simulink model "Proyecto"  (R2023b)
settings: Solver=FixedStepDiscrete  StartTime=0.0  StopTime=100  FixedStep=0.01  MaxStep=0.01  RelTol=1e-3  EnableMultiTasking=on
model workspace (MAT data in the model file):
  d = 0.223
libraries: robotalgslib x1
settings Model: ExtModeTrigDuration=2  Creator=Manuel  LastModifiedBy=Manuel
settings OptimizationCC: EnhancedBackFolding=on  PassReuseOutputArgsAs=Individual arguments  ZeroExternalMemoryAtStartup=off  ZeroInternalMemoryAtStartup=off  MaxStackSize=64  OptimizeBlockOrder=speed  DifferentSizesBufferReuse=on  EfficientTunableParamExpr=on
settings DebuggingCC: AlgebraicLoopMsg=none  ParameterTunabilityLossMsg=error
settings HardwareCC: ProdBitPerInt=16  ProdBitPerPointer=16  ProdBitPerSizeT=16  ProdBitPerPtrDiffT=16  ProdLargestAtomicFloat=None  ProdWordSize=8  ProdHWDeviceType=Atmel->AVR
settings SFSimCC: MATLABDynamicMemAlloc=off
settings RTWCC: Description=Embedded Coder  SystemTargetFile=ert.tlc  HardwareBoard=Arduino Mega 2560  TemplateMakefile=ert_default_tmf  Toolchain=Arduino AVR  BuildConfiguration=Faster Runs
settings CodeAppCC: ForceParamTrailComments=on  IgnoreCustomStorageClasses=off  OperatorAnnotations=on  SimulinkDataObjDesc=on  SFDataObjDesc=on  InsertBlockDesc=on
settings ERTTargetCC: SupportContinuousTime=on  SupportVariableSizeSignals=on  ExtModeTransport=3  ExtModeStaticAlloc=on  ExtModeAutomaticAllocSize=off  ExtModeStaticAllocSize=2048  ExtModeMexFile=ext_xcp  ExtModeIntrfLevel=Level2 - Open

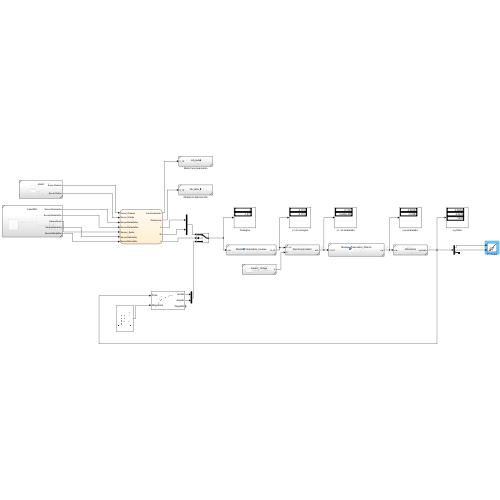
[thumbnail: Simulink's stored preview of the top-level diagram]
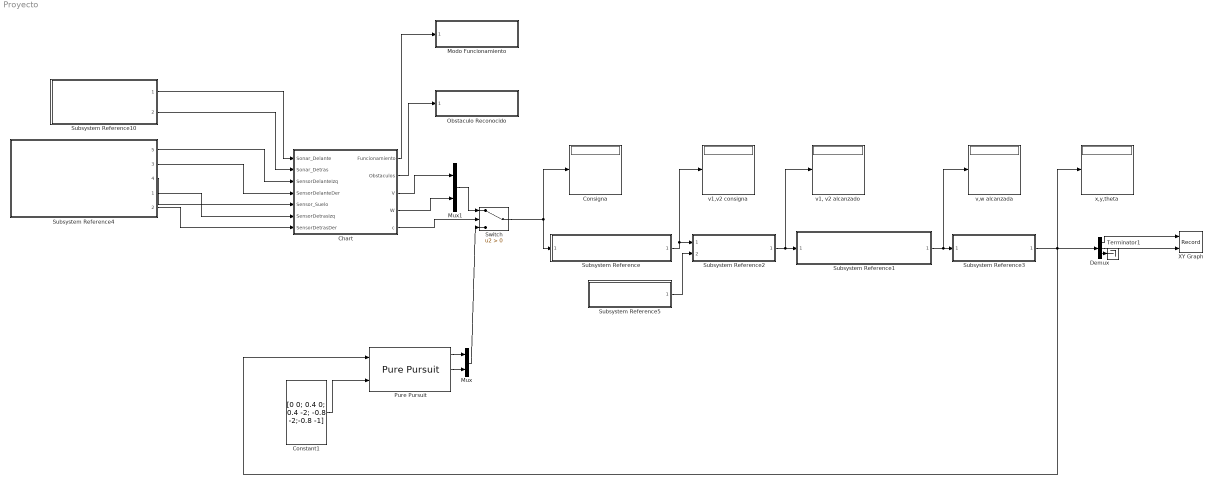
== system Proyecto ==
  Chart : Stateflow chart  TreatAsAtomicUnit=on
      settings: PortSchema="{\"entries\":[{\"content\":{\"sides\":[{\"content\":{\"connectorIds\":[\"In1\",\"In2\",\"In3\",\"In4\",\"In5\",\"In6\",\"In7\"]},\"type\":\"ConnectorPlacement.EquallySpacedRectSide\",\"uuid\":\"4f2d59c3-0ad9-459c-b559-bc93b323e865\"},{\"content\":{\"connectorIds\":[\"Out1\",\"Out2\",\"Out4\",\"Out5\",\"Out3\"],\"side\":\"RIGHT\"},\"type\":\"ConnectorPlacement.EquallySpacedRectSide\",\"uuid\":\"713f980b-cafd-4d08-9887-886c0fa4174d\"},{\"content\":{\"side\":\"TOP\"},\"type\":\"ConnectorPlacement.EquallySpacedRectSide\",\"uuid\":\"6d2f14ce-a548-4b18-94d2-b32a2277c49c\"},{\"content\":{\"side\":\"BOTTOM\"},\"type\":\"ConnectorPlacement.EquallySpacedRectSide\",\"uuid\":\"144d8ec0-92fa-4068-8952-ba018721fcc9\"}]},\"type\":\"ConnectorPlacement.EquallySpacedConnector\",\"uuid\":\"e616e035-6f8b-4bd0-b456-c7d21c102a60\"}],\"packageUris\":[\"http://schema.mathworks.com/mf0/Connector/R2020b\"],\"version\":\"1.0\"}"
  Consigna : Display
  Constant1 : Constant  Value=[0 0; 0.4 0; 0.4 -2; -0.8 -2;-0.8 -1]
  Demux : Demux  Outputs=3
  Modo Funcionamiento : Subsystem  ReferencedSubsystem=Lib_leds
  Mux : Mux  Inputs=2
  Mux1 : Mux  Inputs=2
  Obstaculo Reconocido : Subsystem  ReferencedSubsystem=Lib_leds_2
  Pure Pursuit : robotalgslib/Pure Pursuit  DesiredLinearVelocity=0.3  MaxAngularVelocity=pi/2  LookaheadDistance=0.22  TargetDirPort=on  SimulateUsing=Code generation
      settings: LibrarySourceBlock=navlib/Control Algorithms/Pure Pursuit
  Subsystem Reference : Subsystem  ReferencedSubsystem=Modelo_Cinematico_Inverso
  Subsystem Reference1 : Subsystem  ReferencedSubsystem=Modelo_Cinematico_Directo
  Subsystem Reference10 : Subsystem  ReferencedSubsystem=sonar
  Subsystem Reference2 : Subsystem  ReferencedSubsystem=PieroControladoV
  Subsystem Reference3 : Subsystem  ReferencedSubsystem=Odometria
  Subsystem Reference4 : Subsystem  ReferencedSubsystem=LaserMm
      settings: PortSchema="{\"entries\":[{\"content\":{\"sides\":[{\"content\":{},\"type\":\"ConnectorPlacement.EquallySpacedRectSide\",\"uuid\":\"00a5621a-91c8-4fa0-83fa-79bbc13aa011\"},{\"content\":{\"connectorIds\":[\"Out5\",\"Out3\",\"Out4\",\"Out1\",\"Out2\"],\"side\":\"RIGHT\"},\"type\":\"ConnectorPlacement.EquallySpacedRectSide\",\"uuid\":\"6fca1f99-4dc9-459c-b010-38f5feebdec4\"},{\"content\":{\"side\":\"TOP\"},\"type\":\"ConnectorPlacement.EquallySpacedRectSide\",\"uuid\":\"4ca4df48-19f6-46c7-814a-4f1771035d4e\"}]},\"type\":\"ConnectorPlacement.EquallySpacedConnector\",\"uuid\":\"c2dd7921-69f0-473d-90e2-b93373706358\"}],\"packageUris\":[\"http://schema.mathworks.com/mf0/Connector/R2020b\"],\"version\":\"1.0\"}"
  Subsystem Reference5 : Subsystem  ReferencedSubsystem=Sensor_Voltaje
  Switch : Switch  Criteria=u2 > Threshold  SaturateOnIntegerOverflow=off  InputSameDT=off
  Terminator1 : Terminator
  XY Graph : Record  FileSettingsInternal="{\"entries\":[{\"content\":{\"excelSettings\":{\"content\":{},\"type\":\"Streamout.ExcelSettings\"}},\"type\":\"Streamout.FileSettingStorage\",\"uuid\":\"\"}],\"packageUris\":[\"http:\\/\\/schema.mathworks.com\\/mf0\\/streamout_blocks\\/R2020a\"],\"version\":\"1.0\"}"  Layout=[1 1]  SignalsInternal="{\"entries\":[{\"content\":{\"signals\":[{\"content\":{\"blockPath\":[],\"dimensions\":[1],\"domain\":\"\",\"lineColor\":\"#a2142f\",\"plots\":[1],\"port\":1,\"signalID\":8,\"signalName\":\"Demux:1\"},\"type\":\"RecordBlkView.Signal\",\"uuid\":\"\"},{\"content\":{\"blockPath\":[],\"dimensions\":[1],\"domain\":\"\",\"lineColor\":\"#139fff\",\"plots\":[1],\"port\":2,\"signalID\":11,\"signalName\":\"Demux:2\"},\"type\":\"RecordBlkView.Signal\",\"uuid\":\"\"}]},\"type\":\"RecordBlkView.InputSignals\",\"uuid\":\"\"}],\"packageUris\":[\"http:\\/\\/schema.mathworks.com\\/mf0\\/streamout_blocks\\/R2020a\"],\"version\":\"1.0\"}"  VisualizationBindings="{\"xyplotplugin\":{\"info\":[{\"series\":[{\"bindingParametersList\":[{\"parameter\":\"X-Axis\",\"signalID\":8,\"signalName\":\"Demux:1\"},{\"parameter\":\"Y-Axis\",\"signalID\":11,\"signalName\":\"Demux:2\"}],\"seriesID\":3725}],\"subplotID\":1}]}}"  CompatibilityTag=XY
  "v,w alcanzada " : Display
  "v1, v2 alcanzado" : Display
  v1,v2 consigna : Display
  x,y,theta : Display
  wires:
  Subsystem Reference1/1 -> "v,w alcanzada "/1, Subsystem Reference3/1
  Subsystem Reference/1 -> v1,v2 consigna/1, Subsystem Reference2/1
  Subsystem Reference2/1 -> "v1, v2 alcanzado"/1, Subsystem Reference1/1
  Subsystem Reference3/1 -> x,y,theta/1, Pure Pursuit/1, Demux/1
  Demux/1 -> XY Graph/1
  Demux/2 -> XY Graph/2
  Pure Pursuit/1 -> Mux/1
  Constant1/1 -> Pure Pursuit/2
  Pure Pursuit/2 -> Mux/2
  Switch/1 -> Subsystem Reference/1, Consigna/1
  Mux/1 -> Switch/3
  Chart/3(c) -> Switch/2
  Chart/4(V) -> Mux1/1
  Chart/5(W) -> Mux1/2
  Mux1/1 -> Switch/1
  Subsystem Reference5/1 -> Subsystem Reference2/2
  Demux/3 -> Terminator1/1
  Subsystem Reference10/1 -> Chart/1(Sonar_Delante)
  Subsystem Reference10/2 -> Chart/2(Sonar_Detras)
  Subsystem Reference4/5 -> Chart/3(SensorDelanteIzq)
  Subsystem Reference4/3 -> Chart/4(SensorDelanteDer)
  Subsystem Reference4/4 -> Chart/5(Sensor_Suelo)
  Subsystem Reference4/1 -> Chart/6(SensorDetrasIzq)
  Subsystem Reference4/2 -> Chart/7(SensorDetrasDer)
  Chart/2(Obstaculos) -> Obstaculo Reconocido/1
  Chart/1(Funcionamiento) -> Modo Funcionamiento/1

== stateflow chart Proyecto/Chart ==
  state entrada
    entry:
    V=0;
    W=0;
    c=1;
    Funcionamiento=0;
    Obstaculos=0;
  state Trayectoria
    entry:
    V=0;
    W=0;
    c=0;
    Funcionamiento=2;
    Obstaculos=0;
  state DIzq
    entry:
    V=0.25;
    W=-pi/6;
    c=1;
    Funcionamiento=4;
    Obstaculos=4;
  state DCentro
    entry:
    V=0.1;
    W=-pi/6;
    c=1;
    Funcionamiento=4;
    Obstaculos=8;
  state DDer
    entry:
    V=0.25;
    W=pi/6;
    c=1;
    Funcionamiento=4;
    Obstaculos=2;
  state Caida
    entry:
    V=-0.15;
    W=0;
    c=1;
    Funcionamiento=8;
    Obstaculos=14;
  state Atras_Caida
    entry:
    V=0;
    W=-pi/6;
    c=1;
    Funcionamiento=8;
    Obstaculos=14;
  state Error
    entry:
    V=0;
    W=0;
    c=1;
    Funcionamiento=14;
    Obstaculos=14;
  state DCentroIzq
    entry:
    V=0.1;
    W=-pi/4;
    c=1;
    Funcionamiento=4;
    Obstaculos=5;
  state DCentroDer
    entry:
    V=0.1;
    W=pi/4;
    c=1;
    Funcionamiento=4;
    Obstaculos=3;
  state DTodos
    entry:
    V=0;
    W=-pi/2;
    c=1;
    Funcionamiento=4;
    Obstaculos=9;
  state Atras_Pared
    entry:
    V=-0.2;
    W=-pi/8;
    c=1;
    Funcionamiento=9;
    Obstaculos=0;
  state DIzq1
    entry:
    V=-0.15;
    W=-pi/6;
    c=1;
    Funcionamiento=9;
    Obstaculos=4;
  state DCentro1
    entry:
    V=-0.05;
    W=-pi/6;
    c=1;
    Funcionamiento=9;
    Obstaculos=8;
  state DDer1
    entry:
    V=-0.15;
    W=pi/6;
    c=1;
    Funcionamiento=9;
    Obstaculos=2;
  state DCentroIzq1
    entry:
    V=-0.05;
    W=-pi/4;
    c=1;
    Funcionamiento=9;
    Obstaculos=5;
  state DCentroDer1
    entry:
    V=-0.05;
    W=pi/4;
    c=1;
    Funcionamiento=9;
    Obstaculos=3;
  state DTodos1
    entry:
    V=0;
    W=-pi/2;
    c=1;
    Funcionamiento=9;
    Obstaculos=9;
  (default) -> entrada
  Atras_Caida -> Trayectoria [order 2] : after(3,sec)
  entrada -> Trayectoria : after(2,sec)
  Trayectoria -> Caida [order 1] : [Sensor_Suelo>=10]
  Trayectoria -> DIzq [order 3] : [SensorDelanteIzq<30]
  Trayectoria -> DDer [order 4] : [SensorDelanteDer<30]
  DIzq -> Trayectoria [order 2] : [SensorDelanteIzq>45]
  DCentro -> Trayectoria [order 3] : [Sonar_Delante>45]
  Trayectoria -> DCentro [order 2] : [Sonar_Delante<30]
  DDer -> Trayectoria [order 2] : [SensorDelanteDer>45]
  DCentro -> DCentroIzq [order 2] : [SensorDelanteIzq<30]
  DCentro -> DCentroDer [order 1] : [SensorDelanteDer<30]
  Caida -> Atras_Caida : [Sensor_Suelo<10]
  Atras_Caida -> Error [order 1] : [Sonar_Detras<10 || SensorDetrasDer<10 || SensorDetrasIzq<10]
  DCentroDer -> DCentro [order 3] : [SensorDelanteDer>45]
  DCentroIzq -> DCentro [order 2] : [SensorDelanteIzq>45]
  DCentroIzq -> DIzq [order 3] : [Sonar_Delante>45]
  DIzq -> DCentroIzq [order 1] : [Sonar_Delante<30]
  DDer -> DCentroDer [order 1] : [Sonar_Delante<30]
  DCentroDer -> DDer [order 2] : [Sonar_Delante>45]
  DTodos -> DCentroIzq [order 1] : [SensorDelanteDer>45]
  DCentroIzq -> DTodos [order 1] : [SensorDelanteDer<30]
  DCentroDer -> DTodos [order 1] : [SensorDelanteIzq<30]
  DTodos -> DCentroDer [order 2] : [SensorDelanteIzq>45]
  Atras_Pared -> DTodos [order 1] : [Sonar_Delante>45 || SensorDelanteDer>45 || SensorDelanteIzq>45]
  DTodos -> Atras_Pared [order 3] : [Sonar_Delante<10 || SensorDelanteDer<10 || SensorDelanteIzq<10]
  Atras_Pared -> DDer1 [order 2] : [SensorDetrasDer<30]
  Atras_Pared -> DIzq1 [order 3] : [SensorDetrasIzq<30]
  DIzq1 -> Atras_Pared [order 1] : [SensorDetrasIzq>45]
  DCentro1 -> Atras_Pared [order 3] : [Sonar_Detras>45]
  Atras_Pared -> DCentro1 [order 4] : [Sonar_Detras<30]
  DDer1 -> Atras_Pared [order 2] : [SensorDetrasDer>45]
  DCentro1 -> DCentroIzq1 [order 2] : [SensorDelanteIzq<30]
  DCentro1 -> DCentroDer1 [order 1] : [SensorDetrasDer<30]
  DCentroDer1 -> DCentro1 [order 3] : [SensorDetrasDer>45]
  DCentroIzq1 -> DCentro1 [order 2] : [SensorDetrasIzq>45]
  DCentroIzq1 -> DIzq1 [order 3] : [Sonar_Detras>45]
  DIzq1 -> DCentroIzq1 [order 2] : [Sonar_Detras<30]
  DCentroDer1 -> DDer1 [order 2] : [Sonar_Detras>45]
  DDer1 -> DCentroDer1 [order 1] : [Sonar_Detras<30]
  DTodos1 -> DCentroIzq1 [order 1] : [SensorDetrasDer>45]
  DCentroIzq1 -> DTodos1 [order 1] : [SensorDetrasDer<30]
  DCentroDer1 -> DTodos1 [order 1] : [SensorDetrasIzq<30]
  DTodos1 -> DCentroDer1 [order 2] : [SensorDetrasIzq>45]
  data: Funcionamiento output; Obstaculos output; Sonar_Delante input; Sonar_Detras input; c output; V output double size=1; W output double size=1; SensorDelanteIzq input; SensorDelanteDer input; Sensor_Suelo input; SensorDetrasIzq input; SensorDetrasDer input
